simulink model "Poject_PilotInLoop_Beech_99_Linear_Transfer_Function_Pitch"  (R2018b)
settings: Solver=VariableStepAuto  StartTime=0.0  StopTime=100  RelTol=1e-3
InitFcn:
  | Initial_Data_Pitch
StopFcn:
  | PilotInLoopPlotsPitch
values from neighbouring files (symbols this model uses):
  Kp = -1    [Initial_Data_Pitch.m]    (also in PilotInLoopPitch.m)
  taw = 0.1    [Initial_Data_Pitch.m]    (also in PilotInLoopPitch.m)
  TI = 0.2    [Initial_Data_Pitch.m]    (also in PilotInLoopPitch.m)
  TL = 0.4    [Initial_Data_Pitch.m]    (also in PilotInLoopPitch.m)
  TN = 0.1    [Initial_Data_Pitch.m]    (also in PilotInLoopPitch.m)
settings Model: Creator=User  LastModifiedBy=User

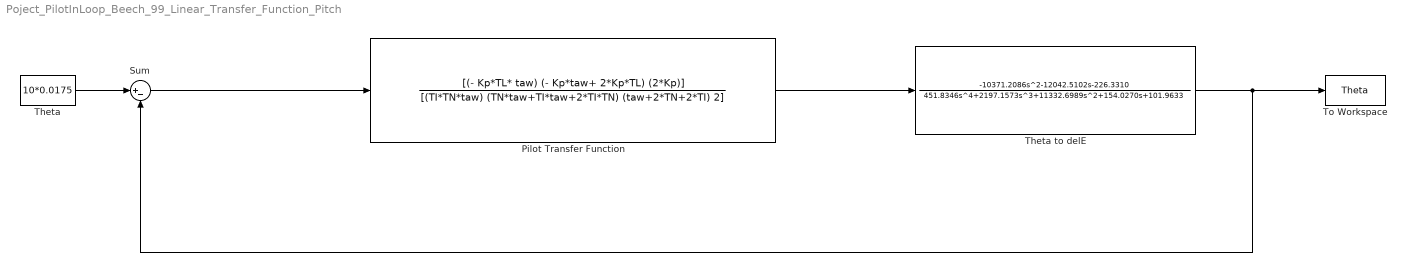
== system Poject_PilotInLoop_Beech_99_Linear_Transfer_Function_Pitch ==
  Pilot Transfer Function : TransferFcn  Numerator=[(- Kp*TL* taw) (- Kp*taw+ 2*Kp*TL) (2*Kp)]  Denominator=[(TI*TN*taw) (TN*taw+TI*taw+2*TI*TN) (taw+2*TN+2*TI) 2]
  Sum : Sum  Inputs=|+-
  Theta : Constant  Value=10*0.0175
  Theta to delE : TransferFcn  Numerator=[-10371.2086 -12042.5102 -226.3310]  Denominator="[451.8346  2197.1573 11332.6989 154.0270 101.9633]"
  To Workspace : ToWorkspace  VariableName=Theta  SaveFormat=Timeseries  SampleTime=-1
  wires:
  Pilot Transfer Function/1 -> Theta to delE/1
  Theta to delE/1 -> To Workspace/1, Sum/2
  Theta/1 -> Sum/1
  Sum/1 -> Pilot Transfer Function/1
